simulink model "y2"  (R2019b)
settings: Solver=VariableStepAuto  StartTime=0.0  StopTime=10.0  RelTol=1e-3
undefined symbols (not defined in the file): ini_y2, ini_y2_d, r2
settings Model: Creator=mic-ciciolla  LastModifiedBy=mic-ciciolla

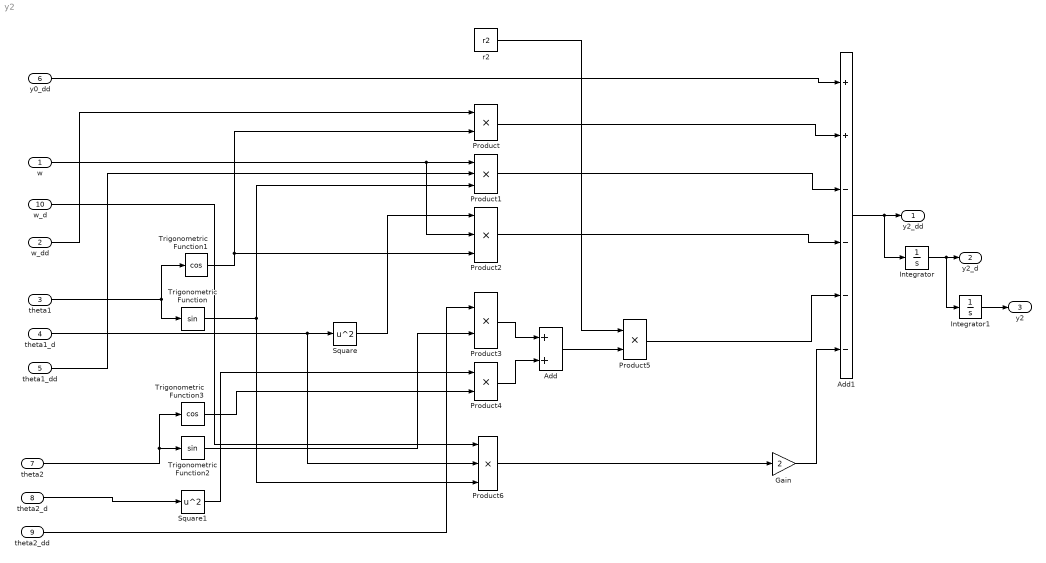
== system y2 ==
  w : Inport
  w_dd : Inport  Port=2
  theta1 : Inport  Port=3
  theta1_d : Inport  Port=4
  theta1_dd : Inport  Port=5
  y0_dd : Inport  Port=6
  theta2 : Inport  Port=7
  theta2_d : Inport  Port=8
  theta2_dd : Inport  Port=9
  w_d : Inport  Port=10
  Add : Sum
  Add1 : Sum  Inputs=++----
  Gain : Gain  Gain=2
  Integrator : Integrator  InitialCondition=ini_y2_d
  Integrator1 : Integrator  InitialCondition=ini_y2
  Product{,3..5} (4 alike) : Product
  Product1 : Product  Inputs=3
  Product2 : Product  Inputs=3
  Product6 : Product  Inputs=3
  Square : Math  Operator=square  SignedPower=off  SaturateOnIntegerOverflow=on
  Square1 : Math  Operator=square  SignedPower=off  SaturateOnIntegerOverflow=on
  Trigonometric Function : Trigonometry
  Trigonometric Function1 : Trigonometry  Operator=cos
  Trigonometric Function2 : Trigonometry
  Trigonometric Function3 : Trigonometry  Operator=cos
  r2 : Constant  Value=r2
  y2_dd : Outport
  y2_d : Outport  Port=2
  y2 : Outport  Port=3
  wires:
  Integrator/1 -> Integrator1/1, y2_d/1
  Integrator1/1 -> y2/1
  Add1/1 -> y2_dd/1, Integrator/1
  y0_dd/1 -> Add1/1
  theta1/1 -> Trigonometric Function1/1, Trigonometric Function/1
  w_dd/1 -> Product/1
  Trigonometric Function1/1 -> Product/2, Product2/3
  Product/1 -> Add1/2
  theta1_dd/1 -> Product1/2
  w/1 -> Product2/2, Product1/1
  Product1/1 -> Add1/3
  Trigonometric Function/1 -> Product1/3, Product6/3
  theta1_d/1 -> Product6/2, Square/1
  Square/1 -> Product2/1
  Product2/1 -> Add1/4
  Product3/1 -> Add/1
  Product4/1 -> Add/2
  Add/1 -> Product5/2
  r2/1 -> Product5/1
  Product5/1 -> Add1/5
  Gain/1 -> Add1/6
  Product6/1 -> Gain/1
  theta2_dd/1 -> Product3/1
  theta2/1 -> Trigonometric Function3/1, Trigonometric Function2/1
  Trigonometric Function2/1 -> Product3/2
  theta2_d/1 -> Square1/1
  Square1/1 -> Product4/1
  Trigonometric Function3/1 -> Product4/2
  w_d/1 -> Product6/1
